simulink model "drone-tp-question4"  (R2025b)
settings: Solver=VariableStepAuto  StartTime=0.0  StopTime=10.0  RelTol=1e-3
values from neighbouring files (symbols this model uses):
  c = (b * sin(alpha)) / m    [drone-tp-observateur-commande.m]
  g = 9.81    [drone-tp-observateur-commande.m]
settings Model: Creator=Etudiant  LastModifiedBy=Etudiant

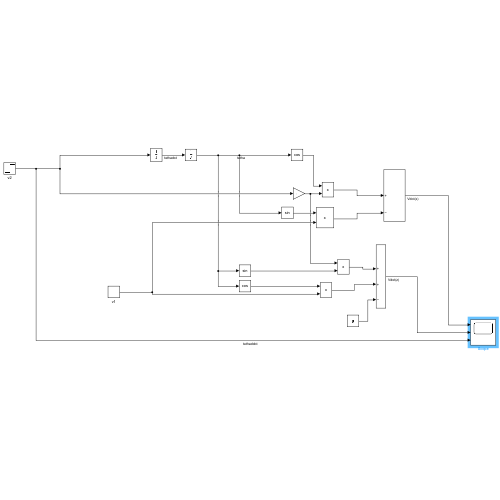
[thumbnail: Simulink's stored preview of the top-level diagram]
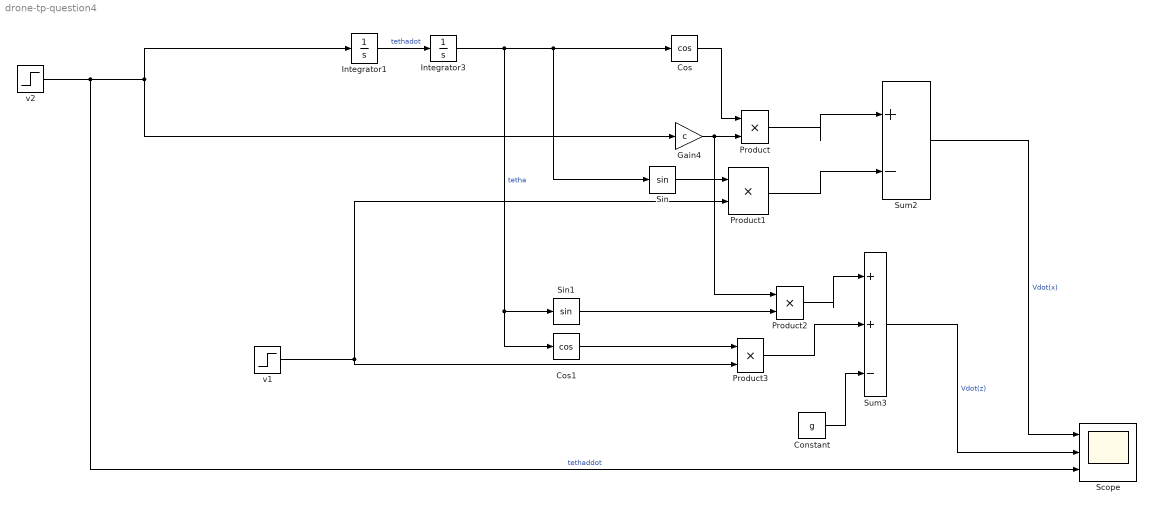
== system drone-tp-question4 ==
  Constant : Constant  Value=g
  Cos : Trigonometry  Operator=cos
  Cos1 : Trigonometry  Operator=cos
  Gain4 : Gain  Gain=c
  Integrator1 : Integrator
  Integrator3 : Integrator  InitialCondition=deg2rad(10)
  Product{,1..3} (4 alike) : Product
  Scope : Scope  NumInputPorts=3
      settings: ActiveDisplayYMinimum=-1.2371665564223298  ActiveDisplayYMaximum=1.2461768468904753
  Sin : Trigonometry
  Sin1 : Trigonometry
  Sum2 : Sum  Inputs=|+-
  Sum3 : Sum  Inputs=|++-
  v1 : Step  SampleTime=0
  v2 : Step  SampleTime=0
  wires:
  v1/1 -> Product3/2, Product1/2
  Sum3/1 -> Scope/2  "Vdot(z)"
  Sum2/1 -> Scope/1  "Vdot(x)"
  Constant/1 -> Sum3/3
  Integrator3/1 -> Sin1/1, Cos1/1, Cos/1, Sin/1  "tetha"
  Product/1 -> Sum2/1
  Product3/1 -> Sum3/2
  v2/1 -> Scope/3, Gain4/1, Integrator1/1  "tethaddot"
  Product2/1 -> Sum3/1
  Cos/1 -> Product/1
  Sin/1 -> Product1/1
  Gain4/1 -> Product2/1, Product/2
  Product1/1 -> Sum2/2
  Integrator1/1 -> Integrator3/1  "tethadot"
  Cos1/1 -> Product3/1
  Sin1/1 -> Product2/2
